simulink model "Fusion_CC_17_reset_clear_read_DTCs_virtual"  (Simulink 9.2)
settings: Solver=VariableStepAuto  StartTime=0.0  StopTime=inf  RelTol=1e-3
undefined symbols (not defined in the file): canChannel
libraries: canlib x3, canmsglib x3
settings Model: Creator=cordunoalbarran  LastModifiedBy=cordunoalbarran
settings DataIOCC: LimitDataPoints=off  SaveFormat=Dataset  SignalLoggingSaveFormat=Dataset
settings OptimizationCC: LifeSpan=auto
settings DebuggingCC: UnderspecifiedInitializationDetection=Simplified  MergeDetectMultiDrivingBlocksExec=error  FcnCallInpInsideContextMsg=error  StateNameClashWarn=none  SFUnexpectedBacktrackingDiag=error  SFNoUnconditionalDefaultTransitionDiag=error  SFExecutionAtInitializationDiag=warning
settings HardwareCC: ProdBitPerPointer=64  ProdBitPerSizeT=64  ProdBitPerPtrDiffT=64  ProdLargestAtomicFloat=Float  ProdIntDivRoundTo=Zero  ProdEndianess=LittleEndian  ProdWordSize=64  ProdHWDeviceType=Intel->x86-64 (Windows64)
settings ModelReferenceCC: PropagateSignalLabelsOutOfModel=on
settings SFSimCC: SimUseLocalCustomCode=on
settings RTWCC: RTWUseLocalCustomCode=on
settings CodeAppCC: StateflowObjectComments=off
settings GRTTargetCC: TargetLangStandard=C99 (ISO)  GeneratePreprocessorConditionals=Use local settings  CombineOutputUpdateFcns=on  GRTInterface=off
settings ConfigComp: CovMetricSettings=dwe  CovHtmlReporting=off  CovSaveCumulativeToWorkspaceVar=off  CovSaveSingleToWorkspaceVar=off  CovExternalEMLEnable=on

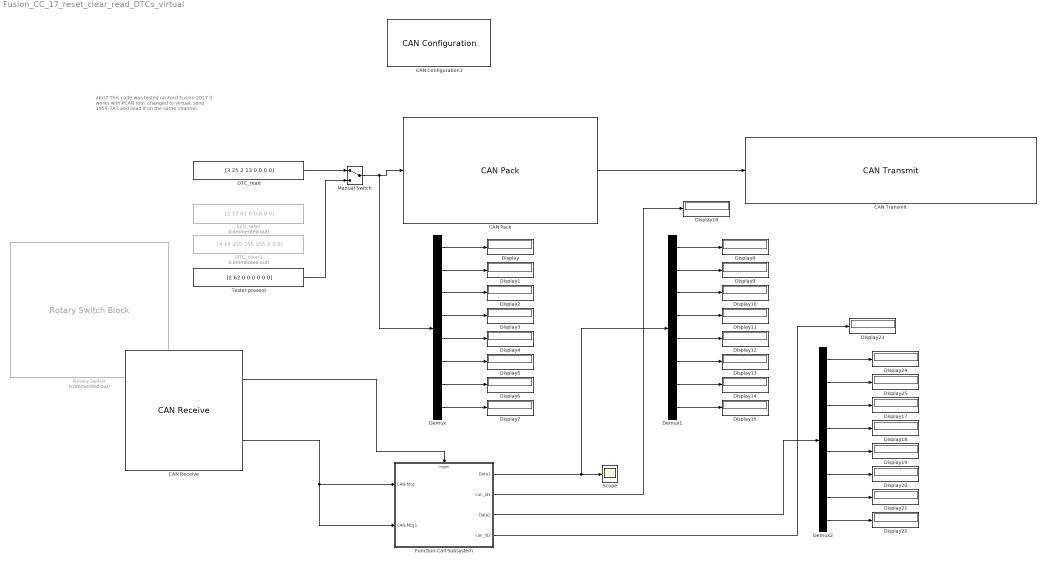
== system Fusion_CC_17_reset_clear_read_DTCs_virtual ==
  note: abr/7 This code was tested on Ford Fusion 2017
      | it works with PCAN tool.
      | changed to virtual.
      | send 1959-7A7 and read it on the same channel.
  CAN Configuration1 : canlib/CAN Configuration  BlockHandle=4.0004  DeviceMenu=MathWorks Virtual 1 (Channel 1)  Device=MathWorks Virtual 1 (Channel 1)  ObjConstructor=canChannel('MathWorks', 'Virtual 1', 1)  BusSpeed=500000  EnableBitParameters=off  AckMode=Normal
      settings: SourceProductName=Vehicle Network Toolbox  SourceProductBaseCode=VN
  CAN Pack : canmsglib/CAN Pack  CANdbFile=C:\Users\cordunoalbarran\Documents\GUv0 Design Docs\CAN\ccan_diagnostic.dbc  MsgList=D_RQ_FUSION_CC  MsgName=D_RQ_FUSION_CC  MsgIDType=Standard (11-bit identifier)  MsgIdentifier=1959  MsgLength=8  SignalInfo=D_RQ_FUSION_CC$56$64$2$2$1$0$1$0$-Inf$Inf$#  NSignals=1  StartBits=str2num('[int32(56)]')  SignalSizes=str2num('[int32(64)]')  ByteOrders=str2num('[int32(2)]')  DataTypes=str2num('[int32(2)]')  MultiplexTypes=str2num('[int32(1)]')  MultiplexValues=str2num('[double(0)]')  Factors=str2num('[double(1)]')  Offsets=str2num('[double(0)]')  Minimums=str2num('[double(-Inf)]')  Maximums=str2num('[double(Inf)]')  Remote=off  ApplyMinMax=off  BusOutput=off
      settings: SourceProductName=Simulink Real-Time  SourceProductBaseCode=XP  DataFormat=raw data
  CAN Receive : canlib/CAN Receive  BlockHandle=6.0004  DeviceMenu=MathWorks Virtual 1 (Channel 1)  Device=MathWorks Virtual 1 (Channel 1)  ObjConstructor=canChannel('MathWorks', 'Virtual 1', 1)  EnableStandardIDsFilter=off  StandardIDs=0  EnableExtendedIDsFilter=off  ExtendedIDs=0  SampleTime=0.01  MsgsPerTimestep=all  StdIDsCombo=Allow all  ExtIDsCombo=Allow all  InternalFilterUpdateStatus=on  BusOutput=off
      settings: SourceProductName=Vehicle Network Toolbox  SourceProductBaseCode=VN
  CAN Transmit : canlib/CAN Transmit  BlockHandle=7.0004  DeviceMenu=MathWorks Virtual 1 (Channel 1)  Device=MathWorks Virtual 1 (Channel 1)  ObjConstructor=canChannel('MathWorks', 'Virtual 1', 1)  EnablePeriodicTransmit=on  MessagePeriod=4
      settings: SourceProductName=Vehicle Network Toolbox  SourceProductBaseCode=VN
  DTC_clear1 : Constant  Commented=on  Value=[4 14 255 255 255 0 0 0]  OutDataTypeStr=uint8  SampleTime=0.01
  DTC_read : Constant  Value=[3 25 2 13 0 0 0 0]  OutDataTypeStr=uint8  SampleTime=0.01
  Demux : Demux  Outputs=8
  Demux1 : Demux  Outputs=8
  Demux2 : Demux  Outputs=8
  Display{,1..25} (26 alike) : Display
  ECU_reset : Constant  Commented=on  Value=[2 17 01 0 0 0 0 0]  OutDataTypeStr=uint8  SampleTime=0.01
  Function-Call Subsystem : Subsystem  TreatAsAtomicUnit=on
  Manual Switch : ManualSwitch
  Rotary Switch : RotarySwitchBlock  Commented=on  WebBlockId=5  Values=DataTag0
  Scope : Scope
  Tester present : Constant  Value=[2 62 0 0 0 0 0 0]  OutDataTypeStr=uint8  SampleTime=0.01
  wires:
  CAN Pack/1 -> CAN Transmit/1
  CAN Receive/2 -> Function-Call Subsystem/2(CAN Msg1), Function-Call Subsystem/1(CAN Msg)
  CAN Receive/1 -> Function-Call Subsystem/Trigger
  Manual Switch/1 -> Demux/1, CAN Pack/1
  DTC_read/1 -> Manual Switch/1
  Demux/1 -> Display/1
  Demux/2 -> Display1/1
  Demux/3 -> Display2/1
  Demux/4 -> Display3/1
  Demux/5 -> Display4/1
  Demux/6 -> Display5/1
  Demux/7 -> Display6/1
  Demux/8 -> Display7/1
  Demux1/8 -> Display15/1
  Demux1/7 -> Display14/1
  Demux1/6 -> Display13/1
  Demux1/5 -> Display12/1
  Demux1/4 -> Display11/1
  Demux1/3 -> Display10/1
  Demux1/2 -> Display9/1
  Demux1/1 -> Display8/1
  Function-Call Subsystem/1(Data1) -> Demux1/1, Scope/1
  Function-Call Subsystem/2(can_id1) -> Display16/1
  Demux2/3 -> Display17/1
  Demux2/2 -> Display25/1
  Demux2/1 -> Display24/1
  Demux2/6 -> Display20/1
  Demux2/8 -> Display22/1
  Demux2/7 -> Display21/1
  Demux2/5 -> Display19/1
  Demux2/4 -> Display18/1
  Function-Call Subsystem/3(Data2) -> Demux2/1
  Function-Call Subsystem/4(can_id2) -> Display23/1
  Tester present/1 -> Manual Switch/2

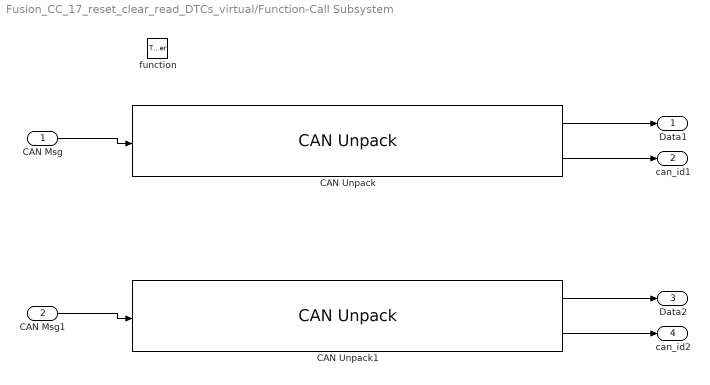
== system Fusion_CC_17_reset_clear_read_DTCs_virtual/Function-Call Subsystem ==
  CAN Msg : Inport
  CAN Msg1 : Inport  Port=2
  function : TriggerPort  TriggerType=function-call  VariantControl=Variant
  CAN Unpack : canmsglib/CAN Unpack  CANdbFile=C:\Users\cordunoalbarran\Documents\GUv0 Design Docs\CAN\ccan_diagnostic.dbc  MsgList=D_RS_FUSION_CC  MsgName=D_RS_FUSION_CC  MsgIDType=Standard (11-bit identifier)  MsgIdentifier=1967  MsgLength=8  SignalInfo=D_RS_FUSION_CC$56$64$2$2$1$0$1$0$-Inf$Inf$#  NSignals=1  IDPort=on  TimestampPort=off  ErrorPort=off  RemotePort=off  LengthPort=off  StatusPort=off  StartBits=str2num('[int32(56)]')  SignalSizes=str2num('[int32(64)]')  ByteOrders=str2num('[int32(2)]')  DataTypes=str2num('[int32(2)]')  MultiplexTypes=str2num('[int32(1)]')  MultiplexValues=str2num('[double(0)]')  Factors=str2num('[double(1)]')  Offsets=str2num('[double(0)]')  Minimums=str2num('[double(-Inf)]')  Maximums=str2num('[double(Inf)]')  ApplyMinMax=off
      settings: SourceProductName=Simulink Real-Time  SourceProductBaseCode=XP  DataFormat=raw data
  CAN Unpack1 : canmsglib/CAN Unpack  CANdbFile=C:\Users\cordunoalbarran\Documents\GUv0 Design Docs\CAN\ccan_diagnostic.dbc  MsgList=D_RQ_FUSION_CC  MsgName=D_RQ_FUSION_CC  MsgIDType=Standard (11-bit identifier)  MsgIdentifier=1959  MsgLength=8  SignalInfo=D_RS_FUSION_CC$56$64$2$2$1$0$1$0$-Inf$Inf$#  NSignals=1  IDPort=on  TimestampPort=off  ErrorPort=off  RemotePort=off  LengthPort=off  StatusPort=off  StartBits=str2num('[int32(56)]')  SignalSizes=str2num('[int32(64)]')  ByteOrders=str2num('[int32(2)]')  DataTypes=str2num('[int32(2)]')  MultiplexTypes=str2num('[int32(1)]')  MultiplexValues=str2num('[double(0)]')  Factors=str2num('[double(1)]')  Offsets=str2num('[double(0)]')  Minimums=str2num('[double(-Inf)]')  Maximums=str2num('[double(Inf)]')  ApplyMinMax=off
      settings: SourceProductName=Simulink Real-Time  SourceProductBaseCode=XP  DataFormat=raw data
  Data1 : Outport
  can_id1 : Outport  Port=2  VectorParamsAs1DForOutWhenUnconnected=on
  Data2 : Outport  Port=3
  can_id2 : Outport  Port=4  VectorParamsAs1DForOutWhenUnconnected=on
  wires:
  CAN Msg/1 -> CAN Unpack/1
  CAN Unpack/1 -> Data1/1
  CAN Unpack/2 -> can_id1/1
  CAN Unpack1/1 -> Data2/1
  CAN Msg1/1 -> CAN Unpack1/1
  CAN Unpack1/2 -> can_id2/1
